simulink model "invpendcart"  (R2021b)
settings: Solver=VariableStepAuto  StartTime=0.0  StopTime=10  RelTol=1e-3
values from neighbouring files (symbols this model uses):
  b = 0.02    [parameter.m]
  g = 9.81    [parameter.m]
  I = 1    [parameter.m]
  kv = 0.02    [parameter.m]
  L = 1.0    (= 1)    [parameter.m]
  M = 6.0    (= 6)    [parameter.m]
  m = 1.5    [parameter.m]
settings Model: Creator=Tolga Catak  LastModifiedBy=Tolga Catak

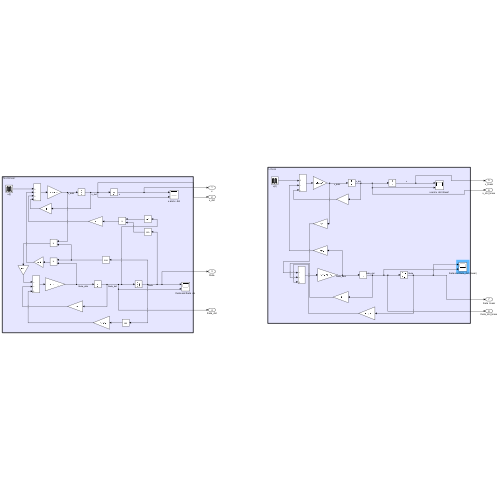
[thumbnail: Simulink's stored preview of the top-level diagram]
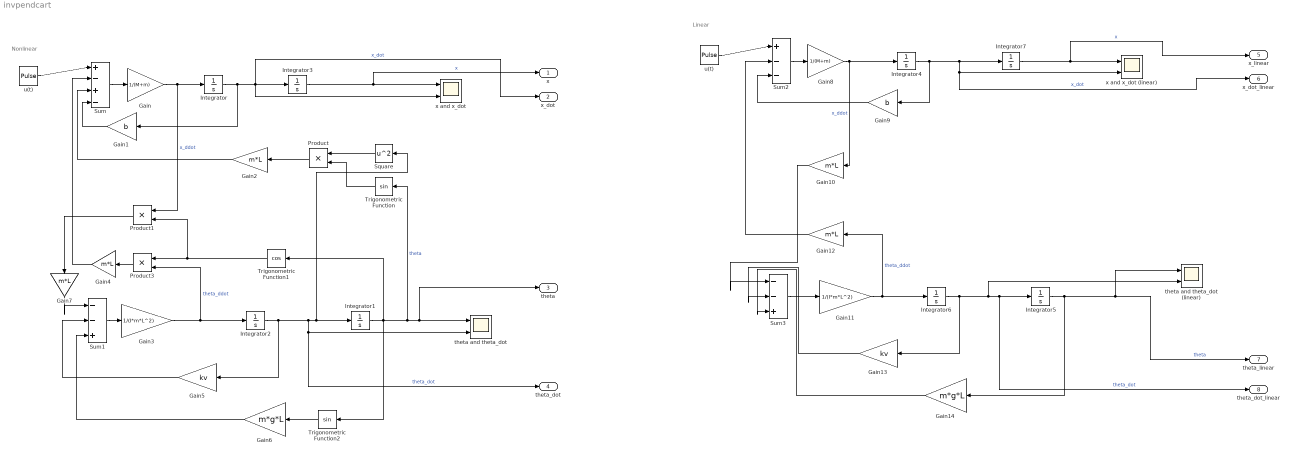
== system invpendcart ==
  note: Linear
  note: Nonlinear
  Gain : Gain  Gain=1/(M+m)
  Gain1 : Gain  Gain=b
  Gain{2,4,7,10,12} (5 alike) : Gain  Gain=m*L
  Gain11 : Gain  Gain=1/(I*m*L^2)
  Gain13 : Gain  Gain=kv
  Gain14 : Gain  Gain=m*g*L
  Gain3 : Gain  Gain=1/(I*m*L^2)
  Gain5 : Gain  Gain=kv
  Gain6 : Gain  Gain=m*g*L
  Gain8 : Gain  Gain=1/(M+m)
  Gain9 : Gain  Gain=b
  Integrator{,2..4,6..7} (6 alike) : Integrator
  Integrator1 : Integrator  LimitOutput=on
  Integrator5 : Integrator  LimitOutput=on
  Product : Product
  Product1 : Product
  Product3 : Product
  Square : Math  Operator=square  SaturateOnIntegerOverflow=on
  Sum : Sum  Inputs=|+-+-
  Sum1 : Sum  Inputs=|--+
  Sum2 : Sum  Inputs=|+--
  Sum3 : Sum  Inputs=|--+
  Trigonometric Function : Trigonometry
  Trigonometric Function1 : Trigonometry  Operator=cos
  Trigonometric Function2 : Trigonometry
  theta and theta_dot : Scope  NumInputPorts=2
  theta and theta_dot (linear) : Scope  NumInputPorts=2
  u(t) : DiscretePulseGenerator  PulseType=Time based  Amplitude=100  Period=100  PulseWidth=0.01
  "u(t) " : DiscretePulseGenerator  PulseType=Time based  Amplitude=100  Period=100  PulseWidth=0.01
  x and x_dot : Scope  NumInputPorts=2
  x and x_dot (linear) : Scope  NumInputPorts=2
  x : Outport
  x_dot : Outport  Port=2
  theta : Outport  Port=3
  theta_dot : Outport  Port=4
  x_linear : Outport  Port=5
  x_dot_linear : Outport  Port=6
  theta_linear : Outport  Port=7
  theta_dot_linear : Outport  Port=8
  wires:
  u(t)/1 -> Sum/1
  Gain5/1 -> Sum1/2
  Gain6/1 -> Sum1/3
  Gain3/1 -> Product3/2, Integrator2/1  "theta_ddot"
  Trigonometric Function2/1 -> Gain6/1
  Sum1/1 -> Gain3/1
  Gain7/1 -> Sum1/1
  Gain4/1 -> Sum/2
  Sum/1 -> Gain/1
  Product3/1 -> Gain4/1
  Product1/1 -> Gain7/1
  Integrator2/1 -> theta_dot/1, theta and theta_dot/2, Square/1, Integrator1/1, Gain5/1  "theta_dot"
  Product/1 -> Gain2/1
  Square/1 -> Product/1
  Trigonometric Function/1 -> Product/2
  Gain1/1 -> Sum/4
  Integrator1/1 -> theta/1, theta and theta_dot/1, Trigonometric Function/1, Trigonometric Function1/1, Trigonometric Function2/1  "theta"
  Integrator/1 -> x and x_dot/2, x_dot/1, Integrator3/1, Gain1/1  "x_dot"
  Trigonometric Function1/1 -> Product1/2, Product3/1
  Integrator3/1 -> x/1, x and x_dot/1  "x"
  Gain/1 -> Product1/1, Integrator/1  "x_ddot"
  Gain2/1 -> Sum/3
  Gain13/1 -> Sum3/2
  "u(t) "/1 -> Sum2/1
  Gain12/1 -> Sum2/2
  Gain9/1 -> Sum2/3
  Sum2/1 -> Gain8/1
  Gain8/1 -> Gain10/1, Integrator4/1  "x_ddot"
  Gain14/1 -> Sum3/3
  Integrator5/1 -> theta_linear/1, theta and theta_dot (linear)/1, Gain14/1  "theta"
  Gain11/1 -> Gain12/1, Integrator6/1  "theta_ddot"
  Gain10/1 -> Sum3/1
  Integrator7/1 -> x_linear/1, x and x_dot (linear)/1  "x"
  Integrator4/1 -> x_dot_linear/1, x and x_dot (linear)/2, Integrator7/1, Gain9/1  "x_dot"
  Integrator6/1 -> theta_dot_linear/1, Integrator5/1, theta and theta_dot (linear)/2, Gain13/1  "theta_dot"
  Sum3/1 -> Gain11/1
